simulink model "impedanceControl_legacy"  (Simulink 8.3)
settings: Solver=FixedStepDiscrete  StartTime=0.0  StopTime=Config.SIMULATION_TIME  FixedStep=Config.Ts  RelTol=1e-3
InitFcn:
  | cd(fileparts(which(bdroot)));
  | initImpedanceControl;
StopFcn:
  | cd(fileparts(which(bdroot)));
  | stopImpedanceControl;
undefined symbols (not defined in the file): AMPLS, Config, FREQS, Kd, Kp, ROBOT_DOF
libraries: WBToolboxLibrary x18
settings Model: Creator=daniele  LastModifiedBy=gnava  CovSFcnEnable=on
settings DebuggingCC: UnderspecifiedInitializationDetection=Simplified  MergeDetectMultiDrivingBlocksExec=error  MultiTaskDSMMsg=warning  MultiTaskCondExecSysMsg=none  FrameProcessingCompatibilityMsg=error  StateNameClashWarn=none  StrictBusMsg=ErrorOnBusTreatedAsVector
settings GRTTargetCC: CombineOutputUpdateFcns=on  GRTInterface=off

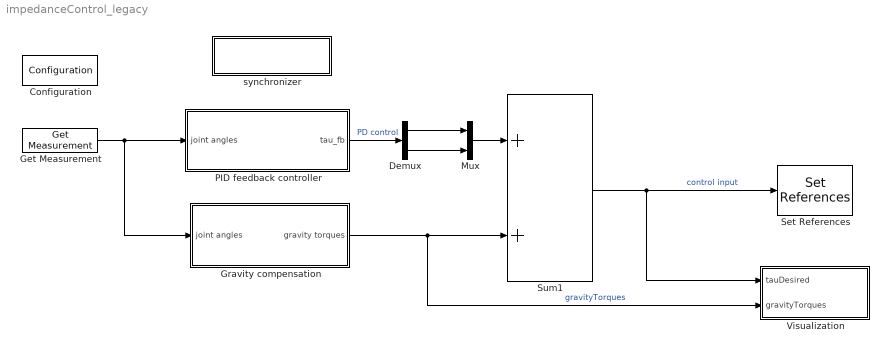
== system impedanceControl_legacy ==
  Configuration : WBToolboxLibrary/Utilities/Configuration  ConfigSource=Workspace  ConfigObject='WBTConfigRobot'  RobotName='icub'  UrdfFile='model.urdf'  ControlledJoints={'l_elbow','l_shoulder_pitch','torso_roll'}  ControlBoardsNames={'left_arm','right_arm','torso'}  LocalName='WBT'  GravityVector=[0,0,-9.81]
  Demux : Demux  Outputs=[11;12]
  Get Measurement : WBToolboxLibrary/wholeBodyStates/Get Measurement  measuredType=Joints Position
  Gravity compensation : Subsystem
  Mux : Mux  Inputs=2
  PID feedback controller : Subsystem
  Set References : WBToolboxLibrary/wholeBodyActuators/Set References  controlType=Torque  refSpeed=50
  Sum1 : Sum
  Visualization : Subsystem
  synchronizer : Subsystem
      mask Display: disp('SYNCHRONIZER')
  wires:
  Get Measurement/1 -> Gravity compensation/1(joint angles), PID feedback controller/1(joint angles)
  Gravity compensation/1(gravity torques) -> Visualization/2(gravityTorques), Sum1/2  "gravityTorques"
  Sum1/1 -> Set References/1, Visualization/1(tauDesired)  "control input"
  PID feedback controller/1(tau_fb) -> Demux/1  "PD control"
  Demux/2 -> Mux/2
  Demux/1 -> Mux/1
  Mux/1 -> Sum1/1

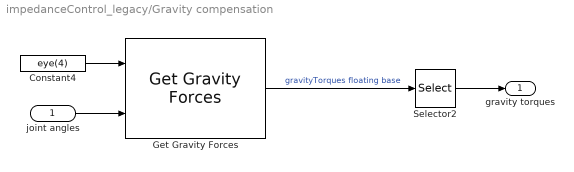
== system impedanceControl_legacy/Gravity compensation ==
  joint angles : Inport
  Constant4 : Constant  Value=eye(4)
  Get Gravity Forces : WBToolboxLibrary/wholeBodyModel/Dynamics/Get Gravity Forces
  Selector2 : Selector  InputPortWidth=ROBOT_DOF+6  IndexOptions=Index vector (dialog)  Indices=[7:ROBOT_DOF+6]  OutputSizes=1
  gravity torques : Outport
  wires:
  Selector2/1 -> gravity torques/1
  Constant4/1 -> Get Gravity Forces/1
  joint angles/1 -> Get Gravity Forces/2
  Get Gravity Forces/1 -> Selector2/1  "gravityTorques floating base"

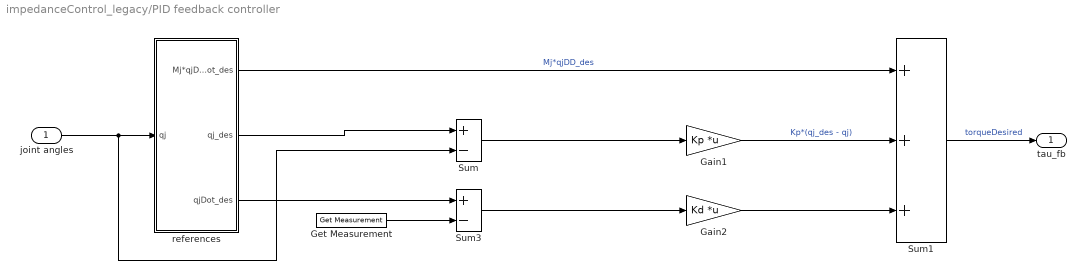
== system impedanceControl_legacy/PID feedback controller ==
  joint angles : Inport
  Gain1 : Gain  Gain=Kp  Multiplication=Matrix(K*u)
  Gain2 : Gain  Gain=Kd  Multiplication=Matrix(K*u)
  Get Measurement : WBToolboxLibrary/wholeBodyStates/Get Measurement  measuredType=Joints Velocity
  Sum : Sum  Inputs=+-
  Sum1 : Sum  Inputs=+++
  Sum3 : Sum  Inputs=+-
  references : Subsystem
  tau_fb : Outport
  wires:
  Get Measurement/1 -> Sum3/2
  Sum/1 -> Gain1/1
  joint angles/1 -> Sum/2, references/1(qj)
  references/1(Mj*qjDDot_des) -> Sum1/1  "Mj*qjDD_des"
  Sum3/1 -> Gain2/1
  references/3(qjDot_des) -> Sum3/1
  Sum1/1 -> tau_fb/1  "torqueDesired"
  references/2(" qj_des") -> Sum/1
  Gain1/1 -> Sum1/2  "Kp*(qj_des - qj)"
  Gain2/1 -> Sum1/3

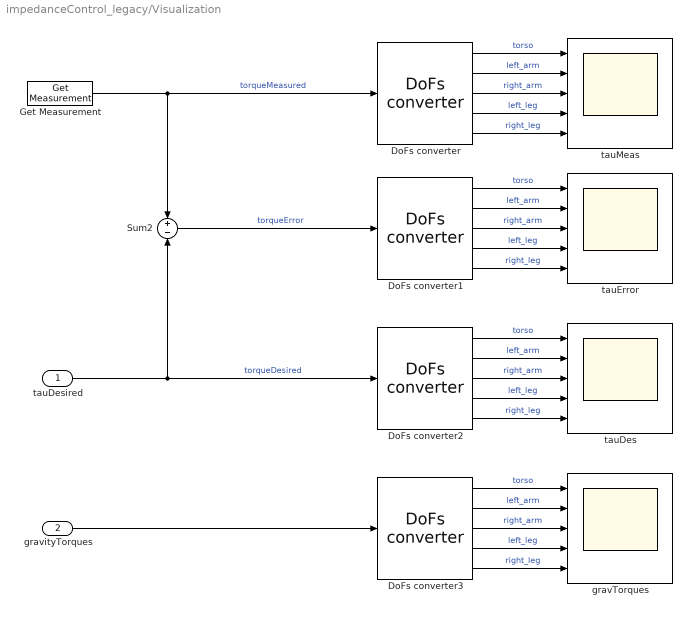
== system impedanceControl_legacy/Visualization ==
  tauDesired : Inport
  gravityTorques : Inport  Port=2
  DoFs converter{,1..3} (4 alike) : WBToolboxLibrary/Utilities/DoFs converter  yarp2WBIOption=From YARP to WBI
  Get Measurement : WBToolboxLibrary/wholeBodyStates/Get Measurement  measuredType=Joints Torque
  Sum2 : Sum  Inputs=+|-
  gravTorques : Scope  NumInputPorts=5
      settings: TimeRange=14  ShowLegends=on  MaxDataPoints=5000  SaveName=gravTorque  YMin=-2.62369~-1.31451~-1.35483~-80.67711~-80.58848  YMax=22.48453~0.36849~0.37657~54.64406~54.86216  SampleTime=-1
  tauDes : Scope  NumInputPorts=5
      settings: TimeRange=14  ShowLegends=on  MaxDataPoints=5000  SaveName=tauDes  YMin=-2.62369~-1.31451~-1.35483~-80.67711~-80.58848  YMax=22.48453~0.36849~0.37657~54.64406~54.86216  SampleTime=-1
  tauError : Scope  NumInputPorts=5
      settings: TimeRange=14  ShowLegends=on  MaxDataPoints=5000  SaveName=tauErr  YMin=-2.62369~-1.31451~-1.35483~-80.67711~-80.58848  YMax=22.48453~0.36849~0.37657~54.64406~54.86216  SampleTime=-1
  tauMeas : Scope  NumInputPorts=5
      settings: TimeRange=14  ShowLegends=on  MaxDataPoints=5000  SaveName=tauMeas  YMin=-2.62369~-1.31451~-1.35483~-80.67711~-80.58848  YMax=22.48453~0.36849~0.37657~54.64406~54.86216  SampleTime=-1
  wires:
  gravityTorques/1 -> DoFs converter3/1
  Get Measurement/1 -> Sum2/1, DoFs converter/1  "torqueMeasured"
  DoFs converter/1 -> tauMeas/1  "torso"
  DoFs converter/2 -> tauMeas/2  "left_arm"
  DoFs converter/4 -> tauMeas/4  "left_leg"
  DoFs converter/3 -> tauMeas/3  "right_arm"
  DoFs converter/5 -> tauMeas/5  "right_leg"
  DoFs converter1/1 -> tauError/1  "torso"
  DoFs converter1/2 -> tauError/2  "left_arm"
  DoFs converter1/4 -> tauError/4  "left_leg"
  DoFs converter1/3 -> tauError/3  "right_arm"
  DoFs converter1/5 -> tauError/5  "right_leg"
  Sum2/1 -> DoFs converter1/1  "torqueError"
  DoFs converter2/1 -> tauDes/1  "torso"
  DoFs converter2/2 -> tauDes/2  "left_arm"
  DoFs converter2/4 -> tauDes/4  "left_leg"
  DoFs converter2/3 -> tauDes/3  "right_arm"
  tauDesired/1 -> DoFs converter2/1, Sum2/2  "torqueDesired"
  DoFs converter2/5 -> tauDes/5  "right_leg"
  DoFs converter3/1 -> gravTorques/1  "torso"
  DoFs converter3/2 -> gravTorques/2  "left_arm"
  DoFs converter3/4 -> gravTorques/4  "left_leg"
  DoFs converter3/3 -> gravTorques/3  "right_arm"
  DoFs converter3/5 -> gravTorques/5  "right_leg"

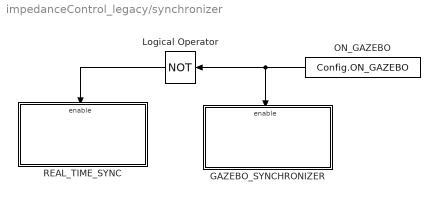
== system impedanceControl_legacy/synchronizer ==
  GAZEBO_SYNCHRONIZER : Subsystem
  Logical Operator : Logic  Operator=NOT  AllPortsSameDT=off  OutDataTypeStr=boolean
  "ON_GAZEBO " : Constant  Value=Config.ON_GAZEBO
  REAL_TIME_SYNC : Subsystem
  wires:
  Logical Operator/1 -> REAL_TIME_SYNC/Enable
  "ON_GAZEBO "/1 -> GAZEBO_SYNCHRONIZER/Enable, Logical Operator/1

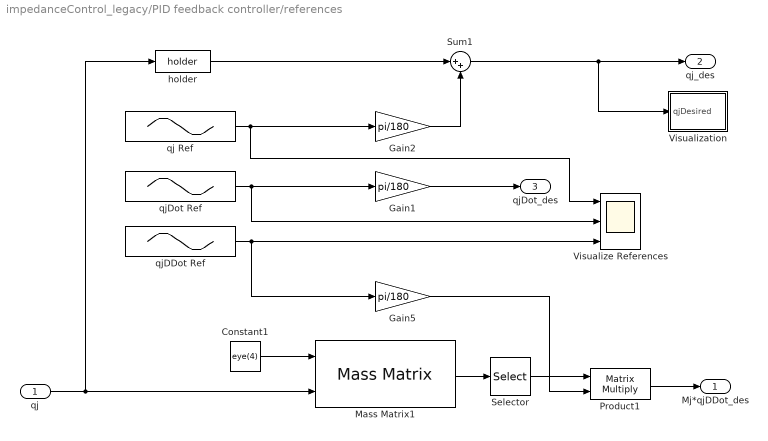
== system impedanceControl_legacy/PID feedback controller/references ==
  qj : Inport
  Constant1 : Constant  Value=eye(4)
  Gain1 : Gain  Gain=pi/180
  Gain2 : Gain  Gain=pi/180
  Gain5 : Gain  Gain=pi/180
  Mass Matrix1 : WBToolboxLibrary/wholeBodyModel/Dynamics/Mass Matrix
  Product1 : Product  Multiplication=Matrix(*)
  Selector : Selector  NumberOfDimensions=2  InputPortWidth=3  IndexOptions=Index vector (dialog),Index vector (dialog)  Indices=[7:ROBOT_DOF+6],[7:ROBOT_DOF+6]  OutputSizes=1,1
  Sum1 : Sum  Inputs=|++
  Visualization : Subsystem
  Visualize References : Scope  NumInputPorts=3
      settings: TimeRange=auto  MaxDataPoints=5000  SaveName=references  YMin=-61.68503~-5~-5  YMax=61.68503~5~5  SampleTime=-1
  holder : WBToolboxLibrary/Utilities/holder 
  qj Ref : Sin  Amplitude=AMPLS  Frequency=FREQS*2*pi  SampleTime=0
  qjDDot Ref : Sin  Amplitude=-AMPLS.*(FREQS*2*pi).^2  Frequency=FREQS*2*pi  SampleTime=0
  qjDot Ref : Sin  Amplitude=AMPLS.*FREQS*2*pi  Frequency=FREQS*2*pi  Phase=pi/2  SampleTime=0
  Mj*qjDDot_des : Outport
  " qj_des" : Outport  Port=2
  qjDot_des : Outport  Port=3
  wires:
  qj Ref/1 -> Visualize References/1, Gain2/1
  qjDot Ref/1 -> Gain1/1, Visualize References/2
  Product1/1 -> Mj*qjDDot_des/1
  Mass Matrix1/1 -> Selector/1
  Selector/1 -> Product1/1
  qjDDot Ref/1 -> Gain5/1, Visualize References/3
  Gain5/1 -> Product1/2
  qj/1 -> holder/1, Mass Matrix1/2
  holder/1 -> Sum1/1
  Constant1/1 -> Mass Matrix1/1
  Gain1/1 -> qjDot_des/1
  Gain2/1 -> Sum1/2
  Sum1/1 -> Visualization/1(qjDesired), " qj_des"/1

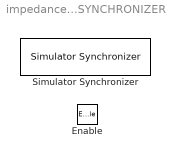
== system impedanceControl_legacy/synchronizer/GAZEBO_SYNCHRONIZER ==
  Enable : EnablePort
  Simulator Synchronizer : WBToolboxLibrary/Utilities/Simulator Synchronizer  period=Config.Ts  serverPortName='/clock/rpc'  clientPortName='/WBT_synchronizer/rpc:o'

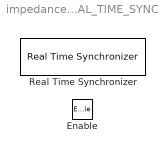
== system impedanceControl_legacy/synchronizer/REAL_TIME_SYNC ==
  Enable : EnablePort
  Real Time Synchronizer : WBToolboxLibrary/Utilities/Real Time Synchronizer  period=Config.Ts

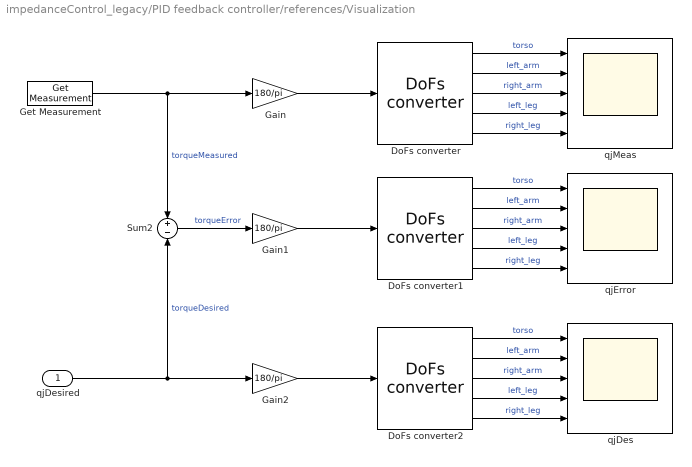
== system impedanceControl_legacy/PID feedback controller/references/Visualization ==
  qjDesired : Inport
  DoFs converter : WBToolboxLibrary/Utilities/DoFs converter  yarp2WBIOption=From YARP to WBI
  DoFs converter1 : WBToolboxLibrary/Utilities/DoFs converter  yarp2WBIOption=From YARP to WBI
  DoFs converter2 : WBToolboxLibrary/Utilities/DoFs converter  yarp2WBIOption=From YARP to WBI
  Gain : Gain  Gain=180/pi
  Gain1 : Gain  Gain=180/pi
  Gain2 : Gain  Gain=180/pi
  Get Measurement : WBToolboxLibrary/wholeBodyStates/Get Measurement  measuredType=Joints Position
  Sum2 : Sum  Inputs=+|-
  qjDes : Scope  NumInputPorts=5
      settings: TimeRange=14  ShowLegends=on  MaxDataPoints=5000  SaveName=qjDes  YMin=-19.45498~-64.64255~-62.0429~-10.72907~-10.51827  YMax=10.88562~67.27378~65.68488~20.79257~18.84043  SampleTime=-1
  qjError : Scope  NumInputPorts=5
      settings: TimeRange=14  ShowLegends=on  MaxDataPoints=5000  SaveName=qjErr  YMin=-2.58811~-2.05965~-1.80349~-9.48486~-9.67523  YMax=2.46722~4.6546~4.43083~9.48486~9.4403  SampleTime=-1
  qjMeas : Scope  NumInputPorts=5
      settings: TimeRange=14  ShowLegends=on  MaxDataPoints=5000  SaveName=qjMeas  YMin=-0.13911~-1.04571~-1.03984~-0.10994~-0.10165  YMax=0.15522~1.32633~1.33197~0.25318~0.23223  SampleTime=-1
  wires:
  Get Measurement/1 -> Sum2/1, Gain/1  "torqueMeasured"
  DoFs converter/1 -> qjMeas/1  "torso"
  DoFs converter/2 -> qjMeas/2  "left_arm"
  DoFs converter/4 -> qjMeas/4  "left_leg"
  DoFs converter/3 -> qjMeas/3  "right_arm"
  DoFs converter/5 -> qjMeas/5  "right_leg"
  DoFs converter1/1 -> qjError/1  "torso"
  DoFs converter1/2 -> qjError/2  "left_arm"
  DoFs converter1/4 -> qjError/4  "left_leg"
  DoFs converter1/3 -> qjError/3  "right_arm"
  DoFs converter1/5 -> qjError/5  "right_leg"
  Sum2/1 -> Gain1/1  "torqueError"
  DoFs converter2/1 -> qjDes/1  "torso"
  DoFs converter2/2 -> qjDes/2  "left_arm"
  DoFs converter2/4 -> qjDes/4  "left_leg"
  DoFs converter2/3 -> qjDes/3  "right_arm"
  qjDesired/1 -> Gain2/1, Sum2/2  "torqueDesired"
  DoFs converter2/5 -> qjDes/5  "right_leg"
  Gain/1 -> DoFs converter/1
  Gain1/1 -> DoFs converter1/1
  Gain2/1 -> DoFs converter2/1
